simulink model "lab1"  (R2024a)
settings: Solver=VariableStepAuto  StartTime=0.0  StopTime=100  MaxStep=1e-2  RelTol=1e-3
values from neighbouring files (symbols this model uses):
  F = 250    [lab_1.m]
  g = 9.81    [lab_1.m]
  k = k_values(i)    [lab_1.m]
  M1 = 150    [lab_1.m]
  M2 = 60    [lab_1.m]
  mu = 0.05    [lab_1.m]
settings Model: Creator=Yoru  LastModifiedBy=Yoru

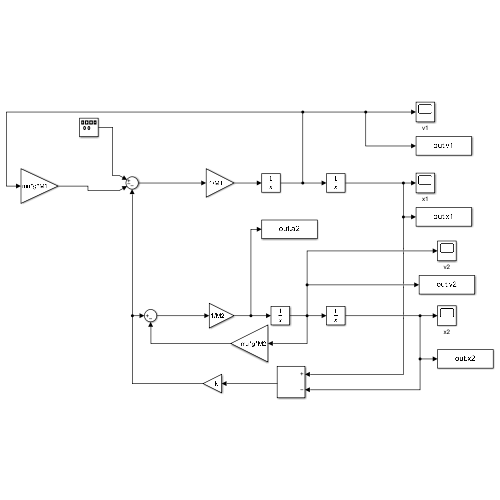
[thumbnail: Simulink's stored preview of the top-level diagram]
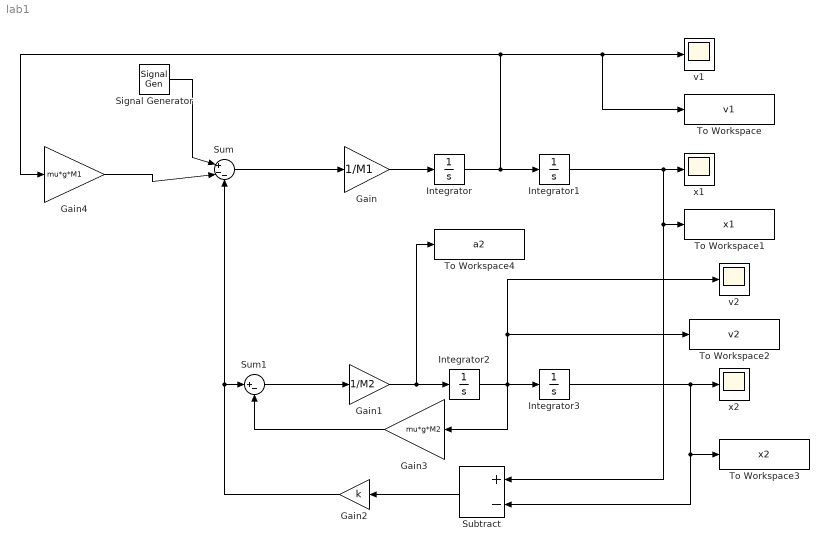
== system lab1 ==
  Gain : Gain  Gain=1/M1
  Gain1 : Gain  Gain=1/M2
  Gain2 : Gain  Gain=k
  Gain3 : Gain  Gain=mu*g*M2
  Gain4 : Gain  Gain=mu*g*M1
  Integrator{,1..3} (4 alike) : Integrator
  Signal Generator : SignalGenerator  WaveForm=square  Amplitude=-F  Frequency=0.01  Units=rad/sec
  Subtract : Sum  Inputs=+-
  Sum : Sum  Inputs=|+--
  Sum1 : Sum  Inputs=|+-
  To Workspace : ToWorkspace  VariableName=v1  SampleTime=-1
  To Workspace1 : ToWorkspace  VariableName=x1  SampleTime=-1
  To Workspace2 : ToWorkspace  VariableName=v2  SampleTime=-1
  To Workspace3 : ToWorkspace  VariableName=x2  SampleTime=-1
  To Workspace4 : ToWorkspace  VariableName=a2  SampleTime=-1
  v1 : Scope
  v2 : Scope
  x1 : Scope
  x2 : Scope
  wires:
  Integrator2/1 -> To Workspace2/1, v2/1, Gain3/1, Integrator3/1
  Gain/1 -> Integrator/1
  Integrator/1 -> Gain4/1, To Workspace/1, v1/1, Integrator1/1
  Integrator1/1 -> Subtract/1, To Workspace1/1, x1/1
  Gain1/1 -> To Workspace4/1, Integrator2/1
  Integrator3/1 -> To Workspace3/1, Subtract/2, x2/1
  Subtract/1 -> Gain2/1
  Gain2/1 -> Sum/3, Sum1/1
  Sum1/1 -> Gain1/1
  Gain3/1 -> Sum1/2
  Signal Generator/1 -> Sum/1
  Sum/1 -> Gain/1
  Gain4/1 -> Sum/2
